simulink library "lib_Axiomatic_Output_Manager"  (R2017a)
settings: Solver=VariableStepAuto  StartTime=0.0  StopTime=10.0  RelTol=1e-3
libraries: simulink x1
settings Model: Creator=Vraj M  LastModifiedBy=Vraj M

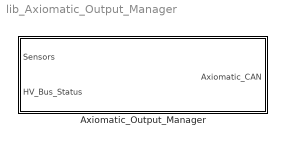
== system lib_Axiomatic_Output_Manager ==
  Axiomatic_Output_Manager : Subsystem

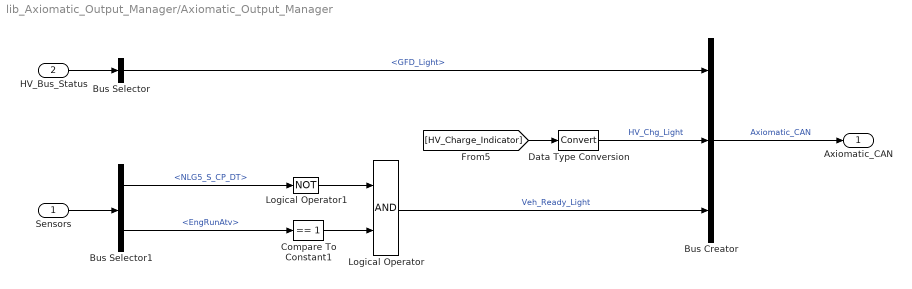
== system lib_Axiomatic_Output_Manager/Axiomatic_Output_Manager ==
  Sensors : Inport
  HV_Bus_Status : Inport  Port=2
  Bus Creator : BusCreator  Inputs=3
  Bus Selector : BusSelector  OutputSignals=GFD_Light
  Bus Selector1 : BusSelector  OutputSignals=from_CAN.fromHV_CAN.from_OBC.NLG5_ST.NLG5_S_CP_DT,from_CAN.fromEBCAN.from_ECM.EngRunAtv
  Compare To Constant1 : simulink/Logic and Bit Operations/Compare To Constant  relop===  const=1  OutDataTypeStr=boolean
  Data Type Conversion : DataTypeConversion
  Logical Operator : Logic  AllPortsSameDT=off  OutDataTypeStr=boolean
  Logical Operator1 : Logic  Operator=NOT  AllPortsSameDT=off  OutDataTypeStr=boolean
  Axiomatic_CAN : Outport
  wires:
  [HV_Charge_Indicator] -> Data Type Conversion/1
  Sensors/1 -> Bus Selector1/1
  Logical Operator/1 -> Bus Creator/3  "Veh_Ready_Light"
  Data Type Conversion/1 -> Bus Creator/2  "HV_Chg_Light"
  Bus Selector/1 -> Bus Creator/1  "<GFD_Light>"
  Bus Creator/1 -> Axiomatic_CAN/1  "Axiomatic_CAN"
  HV_Bus_Status/1 -> Bus Selector/1
  Compare To Constant1/1 -> Logical Operator/2
  Logical Operator1/1 -> Logical Operator/1
  Bus Selector1/2 -> Compare To Constant1/1  "<EngRunAtv>"
  Bus Selector1/1 -> Logical Operator1/1  "<NLG5_S_CP_DT>"
